simulink model "Simulation"  (Simulink 6.0)
settings: Solver=ode3  StartTime=0.0  StopTime=10  FixedStep=5e-3  RelTol=5e-3
libraries: simulink x40, mblibv1 x14, aerolibtransform2 x5, aerolibutil x5
(part 1 of 2)
settings Model: LastModifiedBy=sebastien
settings OptimizationCC: InlineInvariantSignals=off
settings SimMechanicsCC: VisDuringSimulation=on

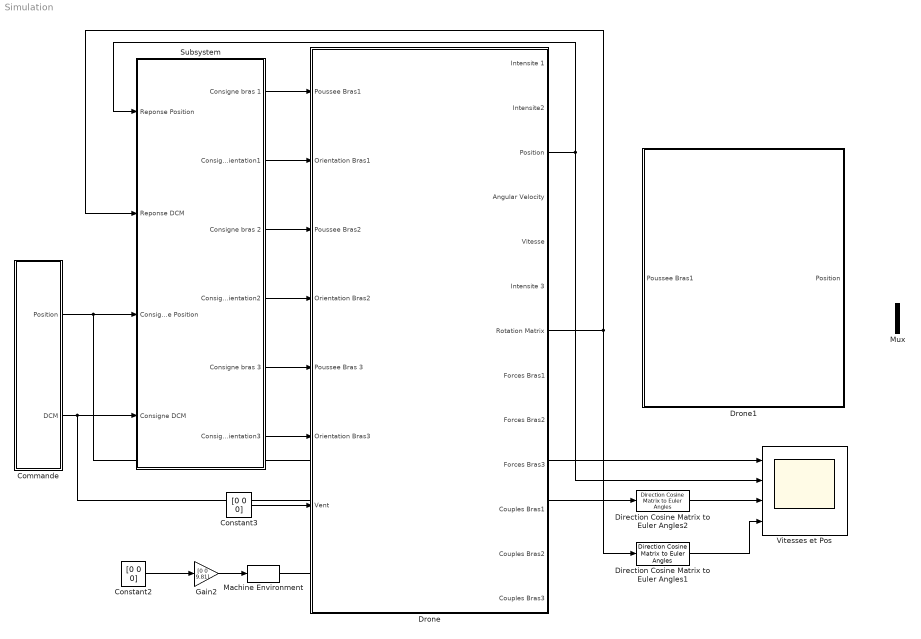
== system Simulation ==
  Commande : Subsystem
  Constant2 : Constant  Value=[0 0 0]
  Constant3 : Constant  Value=[0 0 0]
  Direction Cosine Matrix to Euler Angles1 : aerolibtransform2/Direction Cosine Matrix to Euler Angles
  Direction Cosine Matrix to Euler Angles2 : aerolibtransform2/Direction Cosine Matrix to Euler Angles
  Drone : Subsystem
  Drone1 : Subsystem
  Gain2 : Gain  Gain=[0 0 9.81]
  Machine Environment : mblibv1/Bodies/Machine Environment  Tag=Factory ground  DialogController=MECH.DialogSource  Opaque=on  PortType=env  PhysicalDomain=Mechanical  DialogTemplateClass=MECH.MachineEnvironment  SyncWhenCopied=off  Gravity=[0 0 9.81]  GravityUnits=m/s^2  GravityAsSignal=on  Dimensionality=Auto-detect  AnalysisType=Forward dynamics  LinearAssemblyTolerance=1e-3  LinearAssemblyToleranceUnits=m  AngularAssemblyTolerance=1e-3  AngularAssemblyToleranceUnits=rad  ConstraintSolverType=Stabilizing  ConstraintRelTolerance=1e-4  ConstraintAbsTolerance=1e-4  UseRobustSingularityHandling=off  StatePerturbationType=Fixed  PerturbationSize=1e-5  VisualizeMachine=on
  Mux : Mux  Inputs=2
  Subsystem : Subsystem
  Vitesses et Pos : Scope  NumInputPorts=4
      settings: YMin=-3.5~-45~-9000~-5  YMax=1~5~4000~5  SaveName=ScopeData4
  wires:
  Constant3/1 -> Drone/7(Vent)
  Constant2/1 -> Gain2/1
  Gain2/1 -> Machine Environment/1
  Subsystem/1(Consigne bras 1) -> Drone/1(Poussee Bras1)
  Subsystem/2(Consigne orientation1) -> Drone/2(Orientation Bras1)
  Subsystem/3(Consigne bras 2) -> Drone/3(Poussee Bras2)
  Subsystem/4(Consigne orientation2) -> Drone/4(Orientation Bras2)
  Subsystem/5(Consigne bras 3) -> Drone/5(Poussee Bras 3)
  Subsystem/6(Consigne orientation3) -> Drone/6(Orientation Bras3)
  Drone/7(Rotation Matrix) -> Subsystem/2(Reponse DCM), Direction Cosine Matrix to Euler Angles1/1
  Drone/3(Position) -> Subsystem/1(Reponse Position), Vitesses et Pos/2
  Commande/1(Position) -> Subsystem/3(Consigne Position), Vitesses et Pos/1
  Commande/2(DCM) -> Subsystem/4(Consigne DCM), Direction Cosine Matrix to Euler Angles2/1
  Direction Cosine Matrix to Euler Angles1/1 -> Vitesses et Pos/4
  Direction Cosine Matrix to Euler Angles2/1 -> Vitesses et Pos/3
  connections:
  Drone/LConn1 -- Machine Environment/RConn1

== system Simulation/Commande ==
  Constant : Constant  Value=[0 0 0 0 0 0]
  Demux : Demux  Outputs=2
  Euler Angles to  Direction Cosine Matrix : aerolibtransform2/Euler Angles to  Direction Cosine Matrix
  From File : FromFile  FileName=commande.mat  SampleTime=0
  Reshape1 : simulink/Math Operations/Reshape  OutputDimensionality=1-D array  OutputDimensions=[1,1]
  Reshape2 : simulink/Math Operations/Reshape  OutputDimensionality=1-D array  OutputDimensions=[1,1]
  Reshape3 : simulink/Math Operations/Reshape  OutputDimensionality=1-D array  OutputDimensions=[1,1]
  Position : Outport
  DCM : Outport  Port=2
  wires:
  Reshape2/1 -> Euler Angles to  Direction Cosine Matrix/1
  Reshape3/1 -> Demux/1
  Demux/1 -> Reshape1/1
  Demux/2 -> Reshape2/1
  Reshape1/1 -> Position/1
  From File/1 -> Reshape3/1
  Euler Angles to  Direction Cosine Matrix/1 -> DCM/1

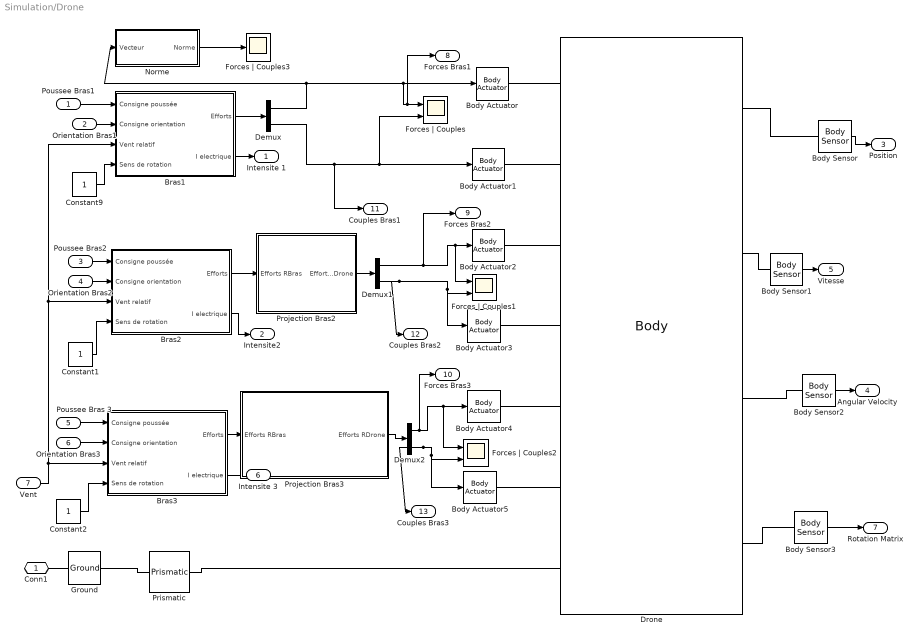
== system Simulation/Drone ==
  Poussee Bras1 : Inport  Port=1  LatchInput=off
  Orientation Bras1 : Inport  Port=2  LatchInput=off
  Poussee Bras2 : Inport  Port=3  LatchInput=off
  Orientation Bras2 : Inport  Port=4  LatchInput=off
  Poussee Bras 3 : Inport  Port=5  LatchInput=off
  Orientation Bras3 : Inport  Port=6  LatchInput=off
  Vent : Inport  Port=7  LatchInput=off
  Body Actuator : mblibv1/Sensors &  Actuators/Body Actuator  Opaque=on  PhysicalDomain=Mechanical  PortType=blob  ActuationStyle=Force  AngleUnits=deg  ArcVelocityUnits=deg/s  ArcAccelerationUnits=deg/s^2  CoordPositionUnits=m  VelocityUnits=m/s  AccelerationUnits=m/s^2  ForceUnits=N  TorqueUnits=N-m  ActiveIO=on  Width=3  DialogClass=MechanicalActuatorBlock  ReferenceFrame=Local (Body CS)  Angle=off  CoordPosition=on  Force=on  Torque=off
  Body Actuator1 : mblibv1/Sensors &  Actuators/Body Actuator  Opaque=on  PhysicalDomain=Mechanical  PortType=blob  ActuationStyle=Force  AngleUnits=deg  ArcVelocityUnits=deg/s  ArcAccelerationUnits=deg/s^2  CoordPositionUnits=m  VelocityUnits=m/s  AccelerationUnits=m/s^2  ForceUnits=N  TorqueUnits=N-m  ActiveIO=on  Width=3  DialogClass=MechanicalActuatorBlock  ReferenceFrame=Local (Body CS)  Angle=off  CoordPosition=on  Force=off  Torque=on
  Body Actuator2 : mblibv1/Sensors &  Actuators/Body Actuator  Opaque=on  PhysicalDomain=Mechanical  PortType=blob  ActuationStyle=Force  AngleUnits=deg  ArcVelocityUnits=deg/s  ArcAccelerationUnits=deg/s^2  CoordPositionUnits=m  VelocityUnits=m/s  AccelerationUnits=m/s^2  ForceUnits=N  TorqueUnits=N-m  ActiveIO=on  Width=3  DialogClass=MechanicalActuatorBlock  ReferenceFrame=Local (Body CS)  Angle=off  CoordPosition=on  Force=on  Torque=off
  Body Actuator3 : mblibv1/Sensors &  Actuators/Body Actuator  Opaque=on  PhysicalDomain=Mechanical  PortType=blob  ActuationStyle=Force  AngleUnits=deg  ArcVelocityUnits=deg/s  ArcAccelerationUnits=deg/s^2  CoordPositionUnits=m  VelocityUnits=m/s  AccelerationUnits=m/s^2  ForceUnits=N  TorqueUnits=N-m  ActiveIO=on  Width=3  DialogClass=MechanicalActuatorBlock  ReferenceFrame=Local (Body CS)  Angle=off  CoordPosition=on  Force=off  Torque=on
  Body Actuator4 : mblibv1/Sensors &  Actuators/Body Actuator  Opaque=on  PhysicalDomain=Mechanical  PortType=blob  ActuationStyle=Force  AngleUnits=deg  ArcVelocityUnits=deg/s  ArcAccelerationUnits=deg/s^2  CoordPositionUnits=m  VelocityUnits=m/s  AccelerationUnits=m/s^2  ForceUnits=N  TorqueUnits=N-m  ActiveIO=on  Width=3  DialogClass=MechanicalActuatorBlock  ReferenceFrame=Local (Body CS)  Angle=off  CoordPosition=on  Force=on  Torque=off
  Body Actuator5 : mblibv1/Sensors &  Actuators/Body Actuator  Opaque=on  PhysicalDomain=Mechanical  PortType=blob  ActuationStyle=Force  AngleUnits=deg  ArcVelocityUnits=deg/s  ArcAccelerationUnits=deg/s^2  CoordPositionUnits=m  VelocityUnits=m/s  AccelerationUnits=m/s^2  ForceUnits=N  TorqueUnits=N-m  ActiveIO=on  Width=3  DialogClass=MechanicalActuatorBlock  ReferenceFrame=Local (Body CS)  Angle=off  CoordPosition=on  Force=off  Torque=on
  Body Sensor : mblibv1/Sensors &  Actuators/Body Sensor  Opaque=on  PhysicalDomain=Mechanical  PortType=blob  Muxed=on  Pose=off  Angle=on  AngleUnits=deg  ArcVelocity=off  ArcVelocityUnits=deg/s  ArcAcceleration=off  ArcAccelerationUnits=deg/s^2  CoordPosition=on  CoordPositionUnits=m  Velocity=off  VelocityUnits=m/s  Acceleration=off  AccelerationUnits=m/s^2  Quaternion=on  QuaternionDT=off  QuaternionDDT=off  OutputVector=[ 3 ]  ActiveIO=on  Width=3  DialogClass=MechanicalSensorBlock  ReferenceFrame=Absolute (World)
  Body Sensor1 : mblibv1/Sensors &  Actuators/Body Sensor  Opaque=on  PhysicalDomain=Mechanical  PortType=blob  Muxed=on  Pose=off  Angle=on  AngleUnits=deg  ArcVelocity=off  ArcVelocityUnits=deg/s  ArcAcceleration=off  ArcAccelerationUnits=deg/s^2  CoordPosition=off  CoordPositionUnits=m  Velocity=on  VelocityUnits=m/s  Acceleration=off  AccelerationUnits=m/s^2  Quaternion=on  QuaternionDT=off  QuaternionDDT=off  QuaternionUnits=off  OutputVector=[ 3 ]  ActiveIO=on  Width=3  DialogClass=MechanicalSensorBlock  ReferenceFrame=Absolute (World)
  Body Sensor2 : mblibv1/Sensors &  Actuators/Body Sensor  Opaque=on  PhysicalDomain=Mechanical  PortType=blob  Muxed=on  Pose=off  Angle=on  AngleUnits=deg  ArcVelocity=on  ArcVelocityUnits=deg/s  ArcAcceleration=off  ArcAccelerationUnits=deg/s^2  CoordPosition=off  CoordPositionUnits=m  Velocity=off  VelocityUnits=m/s  Acceleration=off  AccelerationUnits=m/s^2  Quaternion=on  QuaternionDT=off  QuaternionDDT=off  QuaternionUnits=off  OutputVector=[ 3 ]  ActiveIO=on  Width=3  DialogClass=MechanicalSensorBlock  ReferenceFrame=Absolute (World)
  Body Sensor3 : mblibv1/Sensors &  Actuators/Body Sensor  Opaque=on  PhysicalDomain=Mechanical  PortType=blob  Muxed=on  Pose=on  Angle=on  AngleUnits=deg  ArcVelocity=off  ArcVelocityUnits=deg/s  ArcAcceleration=off  ArcAccelerationUnits=deg/s^2  CoordPosition=off  CoordPositionUnits=m  Velocity=off  VelocityUnits=m/s  Acceleration=off  AccelerationUnits=m/s^2  Quaternion=on  QuaternionDT=off  QuaternionDDT=off  QuaternionUnits=off  OutputVector=[ 9 ]  ActiveIO=on  Width=9  DialogClass=MechanicalSensorBlock  ReferenceFrame=Absolute (World)
  Bras1 : Subsystem
  Bras2 : Subsystem
  Bras3 : Subsystem
  Constant1 : Constant
  Constant2 : Constant
  Constant9 : Constant
  Demux : Demux  Outputs=2
  Demux1 : Demux  Outputs=2
  Demux2 : Demux  Outputs=2
  Drone : mblibv1/Bodies/Body  PhysicalDomain=mechanical  SubClassName=Unknown  LeftPortType=workingframe  RightPortType=workingframe  LConnTagsString=CS3|CS9|CS5|CS10|CS4|CS11|CS1  RConnTagsString=CS2|CS6|CS7|CS8  DialogClass=MechanicalBodyBlock  Mass=1.331  MassUnits=kg  InertiaUnits=kg*m^2  Inertia=[1e-2 9.762e-8 1.027e-6;9.762e-8 0.01 -6.855e-6; 1.027e-6 -6.855e-6 0.018 ]  Shape=Cylinder  ShapeDims=[1 1]  ShapeUnits=m  ShapeUse=false  Density=1  DensityUnits=kg/m^3  DensityUse=false  CG=Left$CG$[0 0 0]$WORLD$WORLD$m$[0 0 0]$Euler X-Y-Z$deg$WORLD$false  WorkingFrames=Right$CS2$[0 0 0]$CG$CG$m$[0 0 0]$Euler X-Y-Z$deg$WORLD$true#Left$CS3$[0.21 0 0]$CG$CG$m$[0 0 0]$Euler X-Y-Z$deg$WORLD$true#Left$CS9$[0.21 0 0]$CG$CG$m$[0 0 0]$Euler X-Y-Z$deg$WORLD$true#Left$CS5$[-0.105 0.1819 0]$CG$CG$m$[0 0 0]$Euler X-Y-Z$deg$WORLD$true#Left$CS10$[-0.105 0.1819 0]$CG$CG$m$[0 0 0]$Euler X-Y-Z$deg$WORLD$true#Left$CS4$[-0.105 -0.1819 0]$CG$CG$m$[0 0 0]$Euler X-Y-Z$deg$WORLD$true#Left$CS11$[-0.105 -0.1819 0]$CG$CG$m$[0 0 0]$Euler X-Y-Z$deg$WORLD$true#Right$CS6$[0 0 0]$CG$CG$m$[0 0 0]$Euler X-Y-Z$deg$WORLD$true#Right$CS7$[0 0 0]$CG$CG$m$[0 0 0]$Euler X-Y-Z$deg$WORLD$true#Right$CS8$[0 0 0]$CG$CG$m$[0 0 0]$Euler X-Y-Z$deg$WORLD$true#Left$CS1$[0 0 0]$CG$CG$m$[0 0 0]$Euler X-Y-Z$deg$WORLD$true
  Forces | Couples : Scope  NumInputPorts=2
      settings: YMin=-6~-1.5  YMax=4~0
  Forces | Couples1 : Scope  NumInputPorts=2
      settings: YMin=-4~-1.25  YMax=0.5~0
  Forces | Couples2 : Scope  NumInputPorts=2
      settings: YMin=-6~-1.5  YMax=1~1.25  SaveName=ScopeData2
  Forces | Couples3 : Scope
      settings: YMin=0  YMax=5.5  SaveName=ScopeData16
  Ground : mblibv1/Bodies/Ground  Opaque=on  LeftPortType=env  RightPortType=workingframe  PhysicalDomain=Mechanical  DialogClass=GroundBlock  CoordPosition=[0 0 0]  CoordPositionUnits=m  StateVectorMgrId=-1  MachineId=[1 0]  ShowEnvPort=on
  Norme : Subsystem  mask{ordre=2}
      mask Display: text(0.3,0.5,strcat('Norme',get_param(gcb, 'ordre')));
  Prismatic : mblibv1/Joints/Prismatic  PhysicalDomain=mechanical  SubClassName=Unknown  LeftPortType=blob  RightPortType=blob  LConnTagsString=__newl0  RConnTagsString=__newr0  NumSAPorts=0  CutJoint=off  MarkAsCut=off  Primitives=prismatic  PrimitiveProps=P1$WORLD$[0 0 1]$prismatic  DialogClass=JointBlock
  Projection Bras2 : Subsystem
  Projection Bras3 : Subsystem
  Conn1 : PMIOPort  Port=1  Side=Left
  Intensite 1 : Outport
  Intensite2 : Outport  Port=2
  Position : Outport  Port=3
  Angular Velocity : Outport  Port=4
  Vitesse : Outport  Port=5
  Intensite 3 : Outport  Port=6
  Rotation Matrix : Outport  Port=7
  Forces Bras1 : Outport  Port=8
  Forces Bras2 : Outport  Port=9
  Forces Bras3 : Outport  Port=10
  Couples Bras1 : Outport  Port=11
  Couples Bras2 : Outport  Port=12
  Couples Bras3 : Outport  Port=13
  wires:
  Bras1/1(Efforts) -> Demux/1
  Demux/1 -> Body Actuator/1, Forces | Couples/1, Forces Bras1/1, Norme/1(Vecteur)
  Demux/2 -> Body Actuator1/1, Forces | Couples/2, Couples Bras1/1
  Bras2/1(Efforts) -> Projection Bras2/1(Efforts RBras)
  Demux1/1 -> Body Actuator2/1, Forces | Couples1/1, Forces Bras2/1
  Demux1/2 -> Body Actuator3/1, Forces | Couples1/2, Couples Bras2/1
  Projection Bras2/1(Efforts RDrone) -> Demux1/1
  Bras3/1(Efforts) -> Projection Bras3/1(Efforts RBras)
  Demux2/1 -> Body Actuator4/1, Forces | Couples2/1, Forces Bras3/1
  Demux2/2 -> Body Actuator5/1, Forces | Couples2/2, Couples Bras3/1
  Projection Bras3/1(Efforts RDrone) -> Demux2/1
  Poussee Bras 3/1 -> Bras3/1(Consigne poussée)
  Constant9/1 -> Bras1/4(Sens de rotation)
  Poussee Bras1/1 -> Bras1/1(Consigne poussée)
  Orientation Bras1/1 -> Bras1/2(Consigne orientation)
  Bras1/2(I electrique) -> Intensite 1/1
  Poussee Bras2/1 -> Bras2/1(Consigne poussée)
  Orientation Bras2/1 -> Bras2/2(Consigne orientation)
  Bras2/2(I electrique) -> Intensite2/1
  Body Sensor/1 -> Position/1
  Body Sensor2/1 -> Angular Velocity/1
  Orientation Bras3/1 -> Bras3/2(Consigne orientation)
  Body Sensor1/1 -> Vitesse/1
  Bras3/2(I electrique) -> Intensite 3/1
  Vent/1 -> Bras1/3(Vent relatif), Bras2/3(Vent relatif), Bras3/3(Vent relatif)
  Body Sensor3/1 -> Rotation Matrix/1
  Constant2/1 -> Bras3/4(Sens de rotation)
  Constant1/1 -> Bras2/4(Sens de rotation)
  Norme/1(Norme) -> Forces | Couples3/1
  connections:
  Body Actuator/RConn1 -- Drone/LConn1
  Body Actuator1/RConn1 -- Drone/LConn2
  Body Actuator2/RConn1 -- Drone/LConn3
  Body Actuator3/RConn1 -- Drone/LConn4
  Body Actuator4/RConn1 -- Drone/LConn5
  Body Actuator5/RConn1 -- Drone/LConn6
  Body Sensor/LConn1 -- Drone/RConn1
  Body Sensor1/LConn1 -- Drone/RConn2
  Drone/RConn3 -- Body Sensor2/LConn1
  Body Sensor3/LConn1 -- Drone/RConn4
  Prismatic/RConn1 -- Drone/LConn7
  Ground/RConn1 -- Prismatic/LConn1
  Conn1/RConn1 -- Ground/LConn1

== system Simulation/Drone1 ==
  Poussee Bras1 : Inport  Port=1  LatchInput=off
  Bras1 : Subsystem  mask{sens=0}
      mask prompts: sens "Sens de rotation"
  Position : Outport

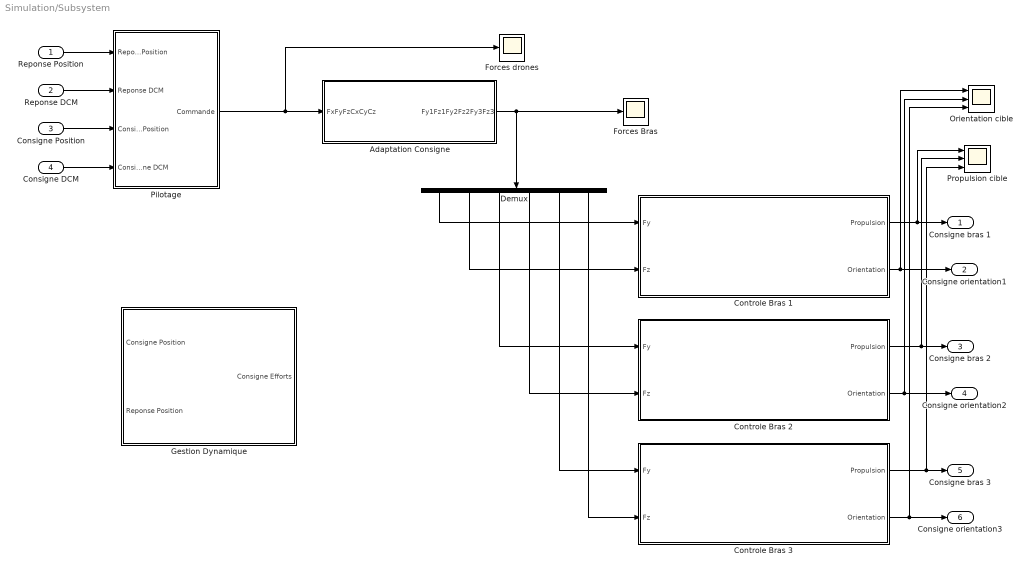
== system Simulation/Subsystem ==
  Reponse Position : Inport  Port=1  LatchInput=off
  Reponse DCM : Inport  Port=2  LatchInput=off
  Consigne Position : Inport  Port=3  LatchInput=off
  Consigne DCM : Inport  Port=4  LatchInput=off
  Adaptation Consigne : Subsystem  mask{l=0.21}
      mask prompts: l "Longueur Bras"
  Controle Bras 1 : Subsystem
  Controle Bras 2 : Subsystem
  Controle Bras 3 : Subsystem
  Demux : Demux  Orientation=down  Outputs=6
  Forces Bras : Scope
      settings: YMin=-0.24  YMax=2.77556e-017  SaveName=ScopeData14
  Forces drones : Scope
      settings: YMin=-0.75  YMax=0  SaveName=ScopeData5
  Gestion Dynamique : Subsystem
  Orientation cible : Scope  NumInputPorts=3
      settings: YMin=-3.5~-5~-5  YMax=3.5~5~5  SaveName=ScopeData15
  Pilotage : Subsystem
  Propulsion cible : Scope  NumInputPorts=3
      settings: YMin=1.9~0~-5  YMax=2.1~2~5  SaveName=ScopeData9
  Consigne bras 1 : Outport
  Consigne orientation1 : Outport  Port=2
  Consigne bras 2 : Outport  Port=3
  Consigne orientation2 : Outport  Port=4
  Consigne bras 3 : Outport  Port=5
  Consigne orientation3 : Outport  Port=6
  wires:
  Pilotage/1(Commande) -> Adaptation Consigne/1(FxFyFzCxCyCz), Forces drones/1
  Reponse Position/1 -> Pilotage/1(Reponse Position)
  Reponse DCM/1 -> Pilotage/2(Reponse DCM)
  Demux/1 -> Controle Bras 1/1(Fy)
  Demux/2 -> Controle Bras 1/2(Fz)
  Adaptation Consigne/1(Fy1Fz1Fy2Fz2Fy3Fz3) -> Demux/1, Forces Bras/1
  Demux/3 -> Controle Bras 2/1(Fy)
  Demux/4 -> Controle Bras 2/2(Fz)
  Demux/5 -> Controle Bras 3/1(Fy)
  Demux/6 -> Controle Bras 3/2(Fz)
  Consigne Position/1 -> Pilotage/3(Consigne Position)
  Consigne DCM/1 -> Pilotage/4(Consigne DCM)
  Controle Bras 1/1(Propulsion) -> Consigne bras 1/1, Propulsion cible/1
  Controle Bras 1/2(Orientation) -> Consigne orientation1/1, Orientation cible/1
  Controle Bras 2/1(Propulsion) -> Consigne bras 2/1, Propulsion cible/2
  Controle Bras 2/2(Orientation) -> Consigne orientation2/1, Orientation cible/2
  Controle Bras 3/1(Propulsion) -> Consigne bras 3/1, Propulsion cible/3
  Controle Bras 3/2(Orientation) -> Consigne orientation3/1, Orientation cible/3

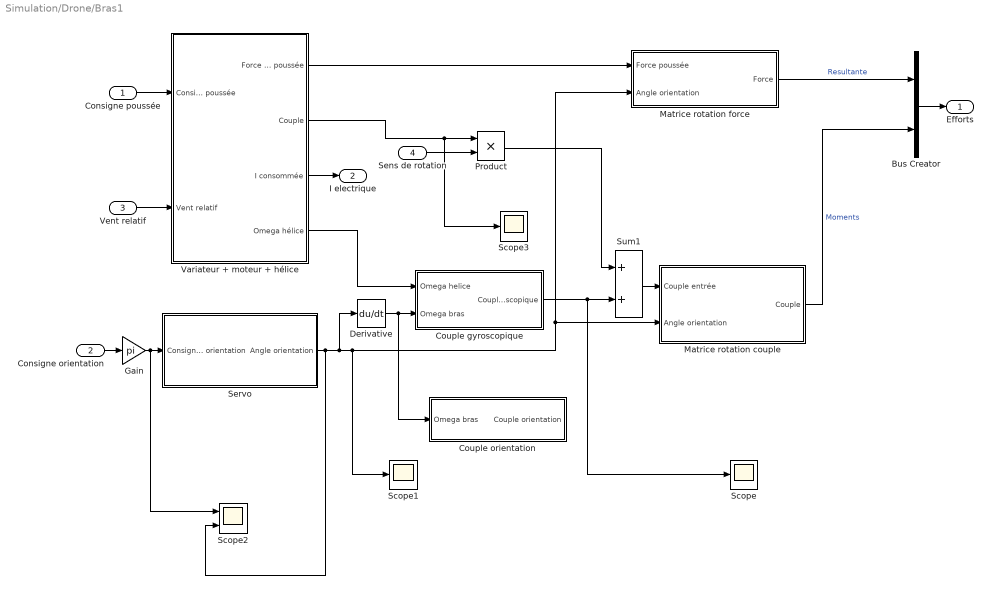
== system Simulation/Drone/Bras1 ==
  Consigne poussée : Inport  Port=1  LatchInput=off
  Consigne orientation : Inport  Port=2  LatchInput=off
  Vent relatif : Inport  Port=3  LatchInput=off
  Sens de rotation : Inport  Port=4  LatchInput=off
  " Couple orientation" : Subsystem
  Bus Creator : BusCreator  DialogController=Simulink.DDGSource_Bus  Inputs=2
  Couple gyroscopique : Subsystem
  Derivative : Derivative
  Gain : Gain  Gain=pi
  Matrice rotation couple : Subsystem
  Matrice rotation force : Subsystem
  Product : Product  RndMeth=Zero
  Scope : Scope
      settings: YMin=-1  YMax=1  SaveName=ScopeData3
  Scope1 : Scope
      settings: YMin=-0.5  YMax=3.75  SaveName=ScopeData8
  Scope2 : Scope  NumInputPorts=2
      settings: YMin=-3~-5  YMax=3~5  SaveName=ScopeData12
  Scope3 : Scope
      settings: YMin=-1  YMax=1  SaveName=ScopeData13
  Servo : Subsystem
  Sum1 : Sum
  Variateur + moteur + hélice : Subsystem
  Efforts : Outport
  I electrique : Outport  Port=2
  wires:
  Consigne poussée/1 -> Variateur + moteur + hélice/1(Consigne poussée)
  Servo/1(Angle orientation) -> Derivative/1, Matrice rotation force/2(Angle orientation), Matrice rotation couple/2(Angle orientation), Scope1/1, Scope2/2
  Matrice rotation force/1(Force) -> Bus Creator/1  "Resultante"
  Matrice rotation couple/1(Couple) -> Bus Creator/2  "Moments"
  Derivative/1 -> Couple gyroscopique/2(Omega bras), " Couple orientation"/1(Omega bras)
  Sum1/1 -> Matrice rotation couple/1(Couple entrée)
  Couple gyroscopique/1(Couple gyroscopique) -> Sum1/2, Scope/1
  Bus Creator/1 -> Efforts/1
  Consigne orientation/1 -> Gain/1
  Vent relatif/1 -> Variateur + moteur + hélice/2(Vent relatif)
  Variateur + moteur + hélice/1(Force de poussée) -> Matrice rotation force/1(Force poussée)
  Variateur + moteur + hélice/3(I consommée) -> I electrique/1
  Variateur + moteur + hélice/4(Omega hélice) -> Couple gyroscopique/1(Omega helice)
  Gain/1 -> Servo/1(Consigne orientation), Scope2/1
  Sens de rotation/1 -> Product/2
  Product/1 -> Sum1/1
  Variateur + moteur + hélice/2(Couple) -> Product/1, Scope3/1

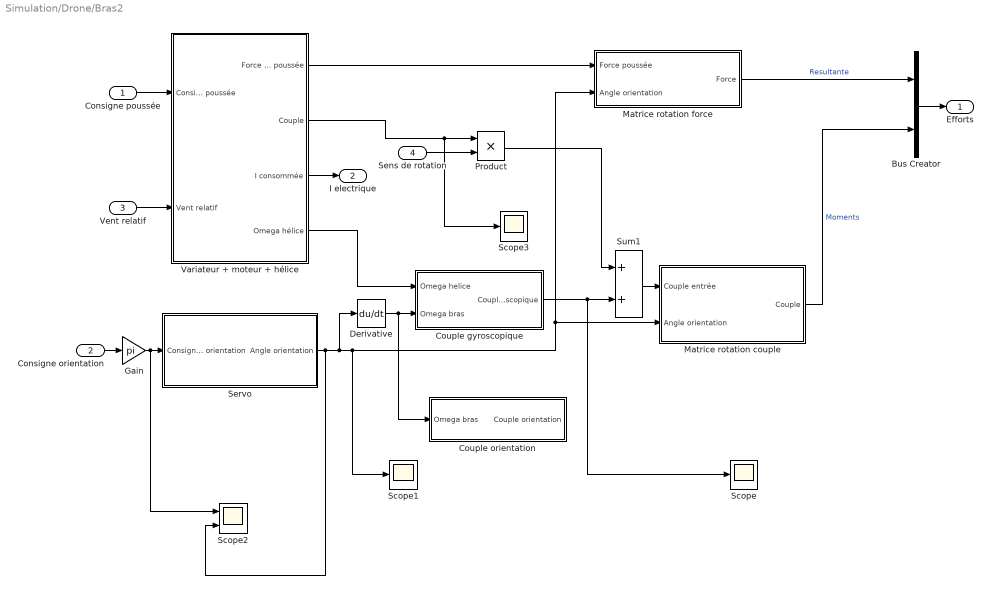
== system Simulation/Drone/Bras2 ==
  Consigne poussée : Inport  Port=1  LatchInput=off
  Consigne orientation : Inport  Port=2  LatchInput=off
  Vent relatif : Inport  Port=3  LatchInput=off
  Sens de rotation : Inport  Port=4  LatchInput=off
  " Couple orientation" : Subsystem
  Bus Creator : BusCreator  DialogController=Simulink.DDGSource_Bus  Inputs=2
  Couple gyroscopique : Subsystem
  Derivative : Derivative
  Gain : Gain  Gain=pi
  Matrice rotation couple : Subsystem
  Matrice rotation force : Subsystem
  Product : Product  RndMeth=Zero
  Scope : Scope
      settings: YMin=-1  YMax=1  SaveName=ScopeData3
  Scope1 : Scope
      settings: YMin=-2.85  YMax=-2.15  SaveName=ScopeData8
  Scope2 : Scope  NumInputPorts=2
      settings: YMin=-3~-5  YMax=3~5  SaveName=ScopeData12
  Scope3 : Scope
      settings: YMin=-1  YMax=1  SaveName=ScopeData13
  Servo : Subsystem
  Sum1 : Sum
  Variateur + moteur + hélice : Subsystem
  Efforts : Outport
  I electrique : Outport  Port=2
  wires:
  Consigne poussée/1 -> Variateur + moteur + hélice/1(Consigne poussée)
  Servo/1(Angle orientation) -> Derivative/1, Matrice rotation force/2(Angle orientation), Matrice rotation couple/2(Angle orientation), Scope1/1, Scope2/2
  Matrice rotation force/1(Force) -> Bus Creator/1  "Resultante"
  Matrice rotation couple/1(Couple) -> Bus Creator/2  "Moments"
  Derivative/1 -> Couple gyroscopique/2(Omega bras), " Couple orientation"/1(Omega bras)
  Sum1/1 -> Matrice rotation couple/1(Couple entrée)
  Couple gyroscopique/1(Couple gyroscopique) -> Sum1/2, Scope/1
  Bus Creator/1 -> Efforts/1
  Consigne orientation/1 -> Gain/1
  Vent relatif/1 -> Variateur + moteur + hélice/2(Vent relatif)
  Variateur + moteur + hélice/1(Force de poussée) -> Matrice rotation force/1(Force poussée)
  Variateur + moteur + hélice/3(I consommée) -> I electrique/1
  Variateur + moteur + hélice/4(Omega hélice) -> Couple gyroscopique/1(Omega helice)
  Gain/1 -> Servo/1(Consigne orientation), Scope2/1
  Sens de rotation/1 -> Product/2
  Product/1 -> Sum1/1
  Variateur + moteur + hélice/2(Couple) -> Product/1, Scope3/1

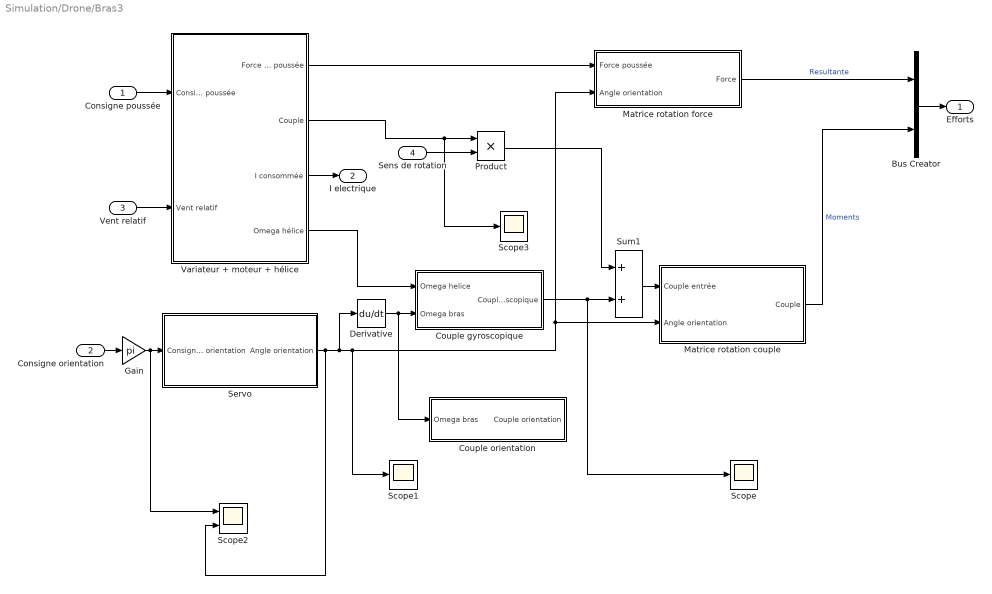
== system Simulation/Drone/Bras3 ==
  Consigne poussée : Inport  Port=1  LatchInput=off
  Consigne orientation : Inport  Port=2  LatchInput=off
  Vent relatif : Inport  Port=3  LatchInput=off
  Sens de rotation : Inport  Port=4  LatchInput=off
  " Couple orientation" : Subsystem
  Bus Creator : BusCreator  DialogController=Simulink.DDGSource_Bus  Inputs=2
  Couple gyroscopique : Subsystem
  Derivative : Derivative
  Gain : Gain  Gain=pi
  Matrice rotation couple : Subsystem
  Matrice rotation force : Subsystem
  Product : Product  RndMeth=Zero
  Scope : Scope
      settings: YMin=-1  YMax=1  SaveName=ScopeData3
  Scope1 : Scope
      settings: YMin=-2.85  YMax=-2.15  SaveName=ScopeData8
  Scope2 : Scope  NumInputPorts=2
      settings: YMin=-3~-5  YMax=3~5  SaveName=ScopeData12
  Scope3 : Scope
      settings: YMin=-1  YMax=1  SaveName=ScopeData13
  Servo : Subsystem
  Sum1 : Sum
  Variateur + moteur + hélice : Subsystem
  Efforts : Outport
  I electrique : Outport  Port=2
  wires:
  Consigne poussée/1 -> Variateur + moteur + hélice/1(Consigne poussée)
  Servo/1(Angle orientation) -> Derivative/1, Matrice rotation force/2(Angle orientation), Matrice rotation couple/2(Angle orientation), Scope1/1, Scope2/2
  Matrice rotation force/1(Force) -> Bus Creator/1  "Resultante"
  Matrice rotation couple/1(Couple) -> Bus Creator/2  "Moments"
  Derivative/1 -> Couple gyroscopique/2(Omega bras), " Couple orientation"/1(Omega bras)
  Sum1/1 -> Matrice rotation couple/1(Couple entrée)
  Couple gyroscopique/1(Couple gyroscopique) -> Sum1/2, Scope/1
  Bus Creator/1 -> Efforts/1
  Consigne orientation/1 -> Gain/1
  Vent relatif/1 -> Variateur + moteur + hélice/2(Vent relatif)
  Variateur + moteur + hélice/1(Force de poussée) -> Matrice rotation force/1(Force poussée)
  Variateur + moteur + hélice/3(I consommée) -> I electrique/1
  Variateur + moteur + hélice/4(Omega hélice) -> Couple gyroscopique/1(Omega helice)
  Gain/1 -> Servo/1(Consigne orientation), Scope2/1
  Sens de rotation/1 -> Product/2
  Product/1 -> Sum1/1
  Variateur + moteur + hélice/2(Couple) -> Product/1, Scope3/1

== system Simulation/Drone/Norme ==
  Vecteur : Inport  Port=1  LatchInput=off
  Constant1 : Constant  Value=ordre
  Math Function : Math  Operator=pow  SaturateOnIntegerOverflow=on
  Math Function1 : Math  Operator=reciprocal  SaturateOnIntegerOverflow=on
  Math Function2 : Math  Operator=pow  SaturateOnIntegerOverflow=on
  Sum of Elements : Sum  Inputs=+  OutScaling=2^-10
  Norme : Outport
  wires:
  Math Function/1 -> Sum of Elements/1
  Vecteur/1 -> Math Function/1
  Constant1/1 -> Math Function/2, Math Function1/1
  Math Function1/1 -> Math Function2/2
  Sum of Elements/1 -> Math Function2/1
  Math Function2/1 -> Norme/1

== system Simulation/Drone/Projection Bras2 ==
  note: Forces
  note: Moments
  Efforts RBras : Inport  Port=1  LatchInput=off
  Bus Creator : BusCreator  DialogController=Simulink.DDGSource_Bus  Inputs=2
  Demux : Demux  Outputs=2
  Gain : Gain  Gain=[cos(2*pi/3) -sin(2*pi/3) 0 ; sin(2*pi/3) cos(2*pi/3) 0; 0 0 1]  Multiplication=Matrix(K*u) (u vector)
  Gain1 : Gain  Gain=[cos(2*pi/3) -sin(2*pi/3) 0 ; sin(2*pi/3) cos(2*pi/3) 0; 0 0 1]  Multiplication=Matrix(K*u) (u vector)
  Efforts RDrone : Outport
  wires:
  Efforts RBras/1 -> Demux/1
  Demux/1 -> Gain/1
  Demux/2 -> Gain1/1
  Bus Creator/1 -> Efforts RDrone/1
  Gain/1 -> Bus Creator/1
  Gain1/1 -> Bus Creator/2

== system Simulation/Drone/Projection Bras3 ==
  note: Forces
  note: Moments
  Efforts RBras : Inport  Port=1  LatchInput=off
  Bus Creator : BusCreator  DialogController=Simulink.DDGSource_Bus  Inputs=2
  Demux : Demux  Outputs=2
  Matrice de Rotation : Gain  Gain=[cos(4*pi/3) -sin(4*pi/3) 0 ; sin(4*pi/3) cos(4*pi/3) 0; 0 0 1]  Multiplication=Matrix(K*u) (u vector)
  "Matrice de rotation " : Gain  Gain=[cos(4*pi/3) -sin(4*pi/3) 0 ; sin(4*pi/3) cos(4*pi/3) 0; 0 0 1]  Multiplication=Matrix(K*u) (u vector)
  Efforts RDrone : Outport
  wires:
  Efforts RBras/1 -> Demux/1
  Demux/1 -> Matrice de Rotation/1
  Demux/2 -> "Matrice de rotation "/1
  Bus Creator/1 -> Efforts RDrone/1
  Matrice de Rotation/1 -> Bus Creator/1
  "Matrice de rotation "/1 -> Bus Creator/2

== system Simulation/Drone1/Bras1 ==
  Consigne poussée : Inport  Port=1  LatchInput=off
  Consigne orientation : Inport  Port=2  LatchInput=off
  Vent relatif : Inport  Port=3  LatchInput=off
  " Couple orientation" : Subsystem
  Bus Creator : BusCreator  DialogController=Simulink.DDGSource_Bus  Inputs=2
  Constant : Constant  Value=sens
  Couple gyroscopique : Subsystem
  Derivative : Derivative
  Gain : Gain  Gain=pi
  Matrice rotation couple : Subsystem
  Matrice rotation force : Subsystem
  Product : Product  RndMeth=Zero
  Servo : Subsystem
  Sum1 : Sum  Inputs=+++
  Variateur + moteur + hélice : Subsystem
  Efforts : Outport
  I electrique : Outport  Port=2
  wires:
  Consigne poussée/1 -> Variateur + moteur + hélice/1(Consigne poussée)
  Servo/1(Angle orientation) -> Derivative/1, Matrice rotation force/2(Angle orientation), Matrice rotation couple/2(Angle orientation)
  Matrice rotation force/1(Force) -> Bus Creator/1  "Resultante"
  Matrice rotation couple/1(Couple) -> Bus Creator/2  "Moments"
  Derivative/1 -> Couple gyroscopique/2(Omega bras), " Couple orientation"/1(Omega bras)
  Sum1/1 -> Matrice rotation couple/1(Couple entrée)
  Couple gyroscopique/1(Couple gyroscopique) -> Sum1/2
  Bus Creator/1 -> Efforts/1
  Consigne orientation/1 -> Gain/1
  Vent relatif/1 -> Variateur + moteur + hélice/2(Vent relatif)
  Variateur + moteur + hélice/1(Force de poussée) -> Matrice rotation force/1(Force poussée)
  Variateur + moteur + hélice/3(I consommée) -> I electrique/1
  Variateur + moteur + hélice/4(Omega hélice) -> Couple gyroscopique/1(Omega helice)
  Gain/1 -> Servo/1(Consigne orientation)
  Constant/1 -> Product/2
  Product/1 -> Sum1/1
  Variateur + moteur + hélice/2(Couple) -> Product/1
  " Couple orientation"/1(Couple orientation) -> Sum1/3

== system Simulation/Subsystem/Adaptation Consigne ==
  FxFyFzCxCyCz : Inport  Port=1  LatchInput=off
  Matrice Correction : Constant  Value=[1 1 1 1/l 1/l 1/l]
  Matrice Transformation : Constant  Value=(1/3)*[0 2 0 0 0 1; 0 0 1 0 2 0; -sqrt(3) -1 0 0 0 1; 0 0 1 -sqrt(3) -1 0; sqrt(3) -1 0 0 0 1; 0 0 1 sqrt(3) -1 0]  VectorParams1D=off
  Product : Product  Multiplication=Matrix(*)  RndMeth=Zero
  Product1 : Product  RndMeth=Zero
  Fy1Fz1Fy2Fz2Fy3Fz3 : Outport
  wires:
  Product/1 -> Fy1Fz1Fy2Fz2Fy3Fz3/1
  Matrice Transformation/1 -> Product/1
  Matrice Correction/1 -> Product1/2
  FxFyFzCxCyCz/1 -> Product1/1
  Product1/1 -> Product/2

== system Simulation/Subsystem/Controle Bras 1 ==
  Fy : Inport  Port=1  LatchInput=off
  Fz : Inport  Port=2  LatchInput=off
  Adaptation Consigne1 : Subsystem  mask{a=2e-5, b=1e-3, c=2e-3}
  Controle Bras1 : Subsystem
  Gain : Gain  Gain=60/(500*2*pi)
  Gain5 : Gain  Gain=1/pi
  Saturation : Saturate  UpperLimit=pi/6  LowerLimit=-pi/6
  Saturation1 : Saturate  UpperLimit=2  LowerLimit=0
  Saturation6 : Saturate  UpperLimit=1000  LowerLimit=0
  Propulsion : Outport
  Orientation : Outport  Port=2
  wires:
  Controle Bras1/1(Force Propulsion) -> Saturation6/1
  Adaptation Consigne1/1(Consigne Omega) -> Gain/1
  Gain/1 -> Saturation1/1
  Saturation6/1 -> Adaptation Consigne1/1(Force)
  Fy/1 -> Controle Bras1/1(Fyc)
  Saturation1/1 -> Propulsion/1
  Fz/1 -> Controle Bras1/2(Fzc)
  Gain5/1 -> Orientation/1
  Controle Bras1/2(Angle Orientation) -> Gain5/1

== system Simulation/Subsystem/Controle Bras 2 ==
  Fy : Inport  Port=1  LatchInput=off
  Fz : Inport  Port=2  LatchInput=off
  Adaptation Consigne1 : Subsystem  mask{a=2e-5, b=1e-3, c=2e-3}
  Controle Bras1 : Subsystem
  Gain : Gain  Gain=60/(500*2*pi)
  Gain5 : Gain  Gain=1/pi
  Saturation1 : Saturate  UpperLimit=2  LowerLimit=0
  Saturation6 : Saturate  UpperLimit=1000  LowerLimit=0
  Propulsion : Outport
  Orientation : Outport  Port=2
  wires:
  Controle Bras1/1(Force Propulsion) -> Saturation6/1
  Adaptation Consigne1/1(Consigne Omega) -> Gain/1
  Gain/1 -> Saturation1/1
  Saturation6/1 -> Adaptation Consigne1/1(Force)
  Fy/1 -> Controle Bras1/1(Fyc)
  Saturation1/1 -> Propulsion/1
  Fz/1 -> Controle Bras1/2(Fzc)
  Gain5/1 -> Orientation/1
  Controle Bras1/2(Angle Orientation) -> Gain5/1

== system Simulation/Subsystem/Controle Bras 3 ==
  Fy : Inport  Port=1  LatchInput=off
  Fz : Inport  Port=2  LatchInput=off
  Adaptation Consigne1 : Subsystem  mask{a=2e-5, b=1e-3, c=2e-3}
  Controle Bras1 : Subsystem
  Gain : Gain  Gain=60/(500*2*pi)
  Gain5 : Gain  Gain=1/pi
  Saturation1 : Saturate  UpperLimit=2  LowerLimit=0
  Saturation6 : Saturate  UpperLimit=1000  LowerLimit=0
  Propulsion : Outport
  Orientation : Outport  Port=2
  wires:
  Controle Bras1/1(Force Propulsion) -> Saturation6/1
  Adaptation Consigne1/1(Consigne Omega) -> Gain/1
  Gain/1 -> Saturation1/1
  Saturation6/1 -> Adaptation Consigne1/1(Force)
  Fy/1 -> Controle Bras1/1(Fyc)
  Saturation1/1 -> Propulsion/1
  Fz/1 -> Controle Bras1/2(Fzc)
  Gain5/1 -> Orientation/1
  Controle Bras1/2(Angle Orientation) -> Gain5/1

== system Simulation/Subsystem/Gestion Dynamique ==
  Consigne Position : Inport  Port=1  LatchInput=off
  Reponse Position : Inport  Port=2  LatchInput=off
  Calcul Position : Subsystem
  Calcul orientation : Subsystem
  PID Attitude : Subsystem  mask{kp=0.00000000001, ki=0, kd=0, kdd=0}
  PID Position : Subsystem  mask{kp=0.5, ki=0.2, kd=2, kdd=0.3}
  Separation composantes : Subsystem
  Separation composantes1 : Subsystem
  Sommation ordres : Subsystem
  Terminator : Terminator
  Consigne Efforts : Outport
  wires:
  Reponse Position/1 -> Separation composantes1/1(Entree), Separation composantes/2(Reponse1)
  Separation composantes1/2(Orientation) -> Calcul Position/2(Orientation), Calcul orientation/2(Orientation)
  Sommation ordres/1(Ordres) -> Consigne Efforts/1
  Separation composantes1/1(Position) -> Terminator/1
  PID Position/1(Sortie) -> Calcul Position/1(Erreur Position)
  Calcul Position/1(Ordres Position) -> Sommation ordres/1(Ordres position)
  Calcul orientation/1(Ordres orientation) -> Sommation ordres/2(Ordres orientation)
  PID Attitude/1(Sortie) -> Calcul orientation/1(Erreur orientation)
  Consigne Position/1 -> Separation composantes/1(Consigne1)
  Separation composantes/1(Erreur Position) -> PID Position/1(Entrée)
  Separation composantes/2(Erreur Attitude) -> PID Attitude/1(Entrée)

== system Simulation/Subsystem/Pilotage ==
  Reponse Position : Inport  Port=1  LatchInput=off
  Reponse DCM : Inport  Port=2  LatchInput=off
  Consigne Position : Inport  Port=3  LatchInput=off
  Consigne DCM : Inport  Port=4  LatchInput=off
  Add : Sum  Inputs=-+  OutScaling=2^-10  InputSameDT=on
  Attitude : Subsystem
  Multiplication : Product  Inputs=**  Multiplication=Matrix(*)  OutScaling=2^-10
  Multiplication1 : Product  Inputs=**  Multiplication=Matrix(*)  OutScaling=2^-10
  Mux1 : Mux  Inputs=2
  PID Attitude : Subsystem  mask{kp=1000, ki=0.05, kd=0.05, kdd=0}
  PID Position : Subsystem  mask{kp=1000, ki=0.05, kd=0.05, kdd=0}
  Commande : Outport
  wires:
  Reponse Position/1 -> Add/1
  Consigne Position/1 -> Add/2
  Add/1 -> PID Position/1(Entrée)
  Consigne DCM/1 -> Attitude/2(Consigne)
  Reponse DCM/1 -> Attitude/1(Reponse), Multiplication1/1, Multiplication/1
  Attitude/1(Commande) -> PID Attitude/1(Entrée)
  PID Attitude/1(Sortie) -> Multiplication/2
  PID Position/1(Sortie) -> Multiplication1/2
  Multiplication1/1 -> Mux1/1
  Multiplication/1 -> Mux1/2
  Mux1/1 -> Commande/1

== system Simulation/Drone/Bras1/ Couple orientation ==
  Omega bras : Inport  Port=1  LatchInput=off
  Derivative1 : Derivative
  Gain : Gain
  Couple orientation : Outport
  wires:
  Omega bras/1 -> Derivative1/1
  Derivative1/1 -> Gain/1
  Gain/1 -> Couple orientation/1

== system Simulation/Drone/Bras1/Couple gyroscopique ==
  Omega helice : Inport  Port=1  LatchInput=off
  Omega bras : Inport  Port=2  LatchInput=off
  Gain : Gain  Gain=[0 27e-6 0]
  Product : Product  RndMeth=Zero
  Couple gyroscopique : Outport
  wires:
  Omega helice/1 -> Product/1
  Omega bras/1 -> Product/2
  Product/1 -> Gain/1
  Gain/1 -> Couple gyroscopique/1

== system Simulation/Drone/Bras1/Matrice rotation couple ==
  Couple entrée : Inport  Port=1  LatchInput=off
  Angle orientation : Inport  Port=2  LatchInput=off
  Constant : Constant  Value=0
  Cos : Trigonometry  Operator=cos
  Gain : Gain  Gain=[ 1 1 -1 ]
  Mux : Mux  Inputs=3
  Product : Product  RndMeth=Zero
  Reshape : simulink/Math Operations/Reshape  OutputDimensionality=1-D array  OutputDimensions=[1,1]
  Sin : Trigonometry
  Couple : Outport
  wires:
  Angle orientation/1 -> Cos/1, Sin/1
  Constant/1 -> Mux/1
  Cos/1 -> Mux/3
  Sin/1 -> Mux/2
  Mux/1 -> Reshape/1
  Gain/1 -> Product/1
  Couple entrée/1 -> Product/2
  Product/1 -> Couple/1
  Reshape/1 -> Gain/1

== system Simulation/Drone/Bras1/Matrice rotation force ==
  Force poussée : Inport  Port=1  LatchInput=off
  Angle orientation : Inport  Port=2  LatchInput=off
  Constant : Constant  Value=0
  Cos : Trigonometry  Operator=cos
  Gain : Gain  Gain=[ 1 1 -1 ]
  Mux : Mux  Inputs=3
  Product : Product  RndMeth=Zero
  Reshape : simulink/Math Operations/Reshape  OutputDimensionality=1-D array  OutputDimensions=[1,1]
  Sin : Trigonometry
  Force : Outport
  wires:
  Angle orientation/1 -> Cos/1, Sin/1
  Constant/1 -> Mux/1
  Cos/1 -> Mux/3
  Sin/1 -> Mux/2
  Mux/1 -> Reshape/1
  Gain/1 -> Product/1
  Force poussée/1 -> Product/2
  Product/1 -> Force/1
  Reshape/1 -> Gain/1

== system Simulation/Drone/Bras1/Servo ==
  Consigne orientation : Inport  Port=1  LatchInput=off
  Temps de réponse orientation1 : TransferFcn  Denominator=[ 0.002 0.05 1]
  Angle orientation : Outport
  wires:
  Consigne orientation/1 -> Temps de réponse orientation1/1
  Temps de réponse orientation1/1 -> Angle orientation/1

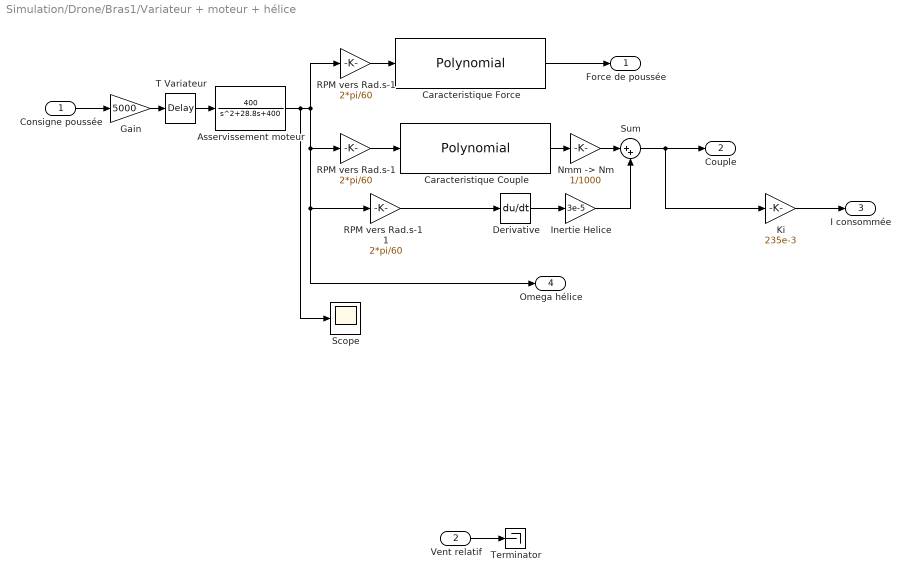
== system Simulation/Drone/Bras1/Variateur + moteur + hélice ==
  Consigne poussée : Inport  Port=1  LatchInput=off
  Vent relatif : Inport  Port=2  LatchInput=off
  Asservissement moteur : TransferFcn  Numerator=[400]  Denominator=[1 28.8 400]
  Caracteristique Couple : simulink/Math Operations/Polynomial  coefs="[3.323e-4  -3.102e-2 1.84e-1]"
  Caracteristique Force : simulink/Math Operations/Polynomial  coefs=[2e-5 -1e-3 2e-3]
  Derivative : Derivative
  Gain : Gain  Gain=5000
  Inertie Helice : Gain  Gain=3e-5
  Ki : Gain  Gain=235e-3
  "Nmm -> Nm" : Gain  Gain=1/1000
  RPM vers Rad.s-1 : Gain  Gain=2*pi/60
  "RPM vers Rad.s-1   " : Gain  Gain=2*pi/60
  RPM vers Rad.s-1   1 : Gain  Gain=2*pi/60
  Scope : Scope
      settings: YMin=4990  YMax=5130  SaveName=ScopeData6
  Sum : Sum  Inputs=|++
  T Variateur : TransportDelay  DelayTime=20e-3
  Terminator : Terminator
  Force de poussée : Outport
  Couple : Outport  Port=2
  I consommée : Outport  Port=3
  Omega hélice : Outport  Port=4
  wires:
  Vent relatif/1 -> Terminator/1
  Consigne poussée/1 -> Gain/1
  Caracteristique Force/1 -> Force de poussée/1
  T Variateur/1 -> Asservissement moteur/1
  Asservissement moteur/1 -> Omega hélice/1, RPM vers Rad.s-1   1/1, "RPM vers Rad.s-1   "/1, RPM vers Rad.s-1/1, Scope/1
  Derivative/1 -> Inertie Helice/1
  Caracteristique Couple/1 -> "Nmm -> Nm"/1
  Sum/1 -> Ki/1, Couple/1
  Inertie Helice/1 -> Sum/2
  Ki/1 -> I consommée/1
  Gain/1 -> T Variateur/1
  RPM vers Rad.s-1/1 -> Caracteristique Force/1
  "RPM vers Rad.s-1   "/1 -> Caracteristique Couple/1
  "Nmm -> Nm"/1 -> Sum/1
  RPM vers Rad.s-1   1/1 -> Derivative/1

== system Simulation/Drone/Bras2/ Couple orientation ==
  Omega bras : Inport  Port=1  LatchInput=off
  Derivative1 : Derivative
  Gain : Gain
  Couple orientation : Outport
  wires:
  Omega bras/1 -> Derivative1/1
  Derivative1/1 -> Gain/1
  Gain/1 -> Couple orientation/1

== system Simulation/Drone/Bras2/Couple gyroscopique ==
  Omega helice : Inport  Port=1  LatchInput=off
  Omega bras : Inport  Port=2  LatchInput=off
  Gain : Gain  Gain=[0 27e-6 0]
  Product : Product  RndMeth=Zero
  Couple gyroscopique : Outport
  wires:
  Omega helice/1 -> Product/1
  Omega bras/1 -> Product/2
  Product/1 -> Gain/1
  Gain/1 -> Couple gyroscopique/1

== system Simulation/Drone/Bras2/Matrice rotation couple ==
  Couple entrée : Inport  Port=1  LatchInput=off
  Angle orientation : Inport  Port=2  LatchInput=off
  Constant : Constant  Value=0
  Cos : Trigonometry  Operator=cos
  Gain : Gain  Gain=[ 1 1 -1 ]
  Mux : Mux  Inputs=3
  Product : Product  RndMeth=Zero
  Reshape : simulink/Math Operations/Reshape  OutputDimensionality=1-D array  OutputDimensions=[1,1]
  Sin : Trigonometry
  Couple : Outport
  wires:
  Angle orientation/1 -> Cos/1, Sin/1
  Constant/1 -> Mux/1
  Cos/1 -> Mux/3
  Sin/1 -> Mux/2
  Mux/1 -> Reshape/1
  Gain/1 -> Product/1
  Couple entrée/1 -> Product/2
  Product/1 -> Couple/1
  Reshape/1 -> Gain/1

== system Simulation/Drone/Bras2/Matrice rotation force ==
  Force poussée : Inport  Port=1  LatchInput=off
  Angle orientation : Inport  Port=2  LatchInput=off
  Constant : Constant  Value=0
  Cos : Trigonometry  Operator=cos
  Gain : Gain  Gain=[ 1 1 -1 ]
  Mux : Mux  Inputs=3
  Product : Product  RndMeth=Zero
  Reshape : simulink/Math Operations/Reshape  OutputDimensionality=1-D array  OutputDimensions=[1,1]
  Sin : Trigonometry
  Force : Outport
  wires:
  Angle orientation/1 -> Cos/1, Sin/1
  Constant/1 -> Mux/1
  Cos/1 -> Mux/3
  Sin/1 -> Mux/2
  Mux/1 -> Reshape/1
  Gain/1 -> Product/1
  Force poussée/1 -> Product/2
  Product/1 -> Force/1
  Reshape/1 -> Gain/1

== system Simulation/Drone/Bras2/Servo ==
  Consigne orientation : Inport  Port=1  LatchInput=off
  Temps de réponse orientation1 : TransferFcn  Denominator=[ 0.002 0.05 1]
  Angle orientation : Outport
  wires:
  Consigne orientation/1 -> Temps de réponse orientation1/1
  Temps de réponse orientation1/1 -> Angle orientation/1

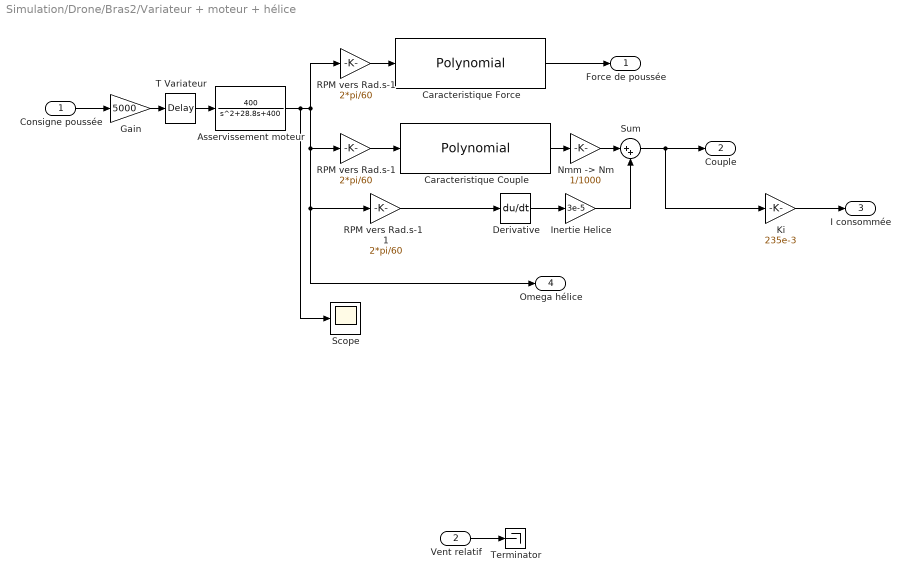
== system Simulation/Drone/Bras2/Variateur + moteur + hélice ==
  Consigne poussée : Inport  Port=1  LatchInput=off
  Vent relatif : Inport  Port=2  LatchInput=off
  Asservissement moteur : TransferFcn  Numerator=[400]  Denominator=[1 28.8 400]
  Caracteristique Couple : simulink/Math Operations/Polynomial  coefs="[3.323e-4  -3.102e-2 1.84e-1]"
  Caracteristique Force : simulink/Math Operations/Polynomial  coefs=[2e-5 -1e-3 2e-3]
  Derivative : Derivative
  Gain : Gain  Gain=5000
  Inertie Helice : Gain  Gain=3e-5
  Ki : Gain  Gain=235e-3
  "Nmm -> Nm" : Gain  Gain=1/1000
  RPM vers Rad.s-1 : Gain  Gain=2*pi/60
  "RPM vers Rad.s-1   " : Gain  Gain=2*pi/60
  RPM vers Rad.s-1   1 : Gain  Gain=2*pi/60
  Scope : Scope
      settings: YMin=4990  YMax=5130  SaveName=ScopeData6
  Sum : Sum  Inputs=|++
  T Variateur : TransportDelay  DelayTime=20e-3
  Terminator : Terminator
  Force de poussée : Outport
  Couple : Outport  Port=2
  I consommée : Outport  Port=3
  Omega hélice : Outport  Port=4
  wires:
  Vent relatif/1 -> Terminator/1
  Consigne poussée/1 -> Gain/1
  Caracteristique Force/1 -> Force de poussée/1
  T Variateur/1 -> Asservissement moteur/1
  Asservissement moteur/1 -> Omega hélice/1, RPM vers Rad.s-1   1/1, "RPM vers Rad.s-1   "/1, RPM vers Rad.s-1/1, Scope/1
  Derivative/1 -> Inertie Helice/1
  Caracteristique Couple/1 -> "Nmm -> Nm"/1
  Sum/1 -> Ki/1, Couple/1
  Inertie Helice/1 -> Sum/2
  Ki/1 -> I consommée/1
  Gain/1 -> T Variateur/1
  RPM vers Rad.s-1/1 -> Caracteristique Force/1
  "RPM vers Rad.s-1   "/1 -> Caracteristique Couple/1
  "Nmm -> Nm"/1 -> Sum/1
  RPM vers Rad.s-1   1/1 -> Derivative/1

== system Simulation/Drone/Bras3/ Couple orientation ==
  Omega bras : Inport  Port=1  LatchInput=off
  Derivative1 : Derivative
  Gain : Gain
  Couple orientation : Outport
  wires:
  Omega bras/1 -> Derivative1/1
  Derivative1/1 -> Gain/1
  Gain/1 -> Couple orientation/1

== system Simulation/Drone/Bras3/Couple gyroscopique ==
  Omega helice : Inport  Port=1  LatchInput=off
  Omega bras : Inport  Port=2  LatchInput=off
  Gain : Gain  Gain=[0 27e-6 0]
  Product : Product  RndMeth=Zero
  Couple gyroscopique : Outport
  wires:
  Omega helice/1 -> Product/1
  Omega bras/1 -> Product/2
  Product/1 -> Gain/1
  Gain/1 -> Couple gyroscopique/1

== system Simulation/Drone/Bras3/Matrice rotation couple ==
  Couple entrée : Inport  Port=1  LatchInput=off
  Angle orientation : Inport  Port=2  LatchInput=off
  Constant : Constant  Value=0
  Cos : Trigonometry  Operator=cos
  Gain : Gain  Gain=[ 1 1 -1 ]
  Mux : Mux  Inputs=3
  Product : Product  RndMeth=Zero
  Reshape : simulink/Math Operations/Reshape  OutputDimensionality=1-D array  OutputDimensions=[1,1]
  Sin : Trigonometry
  Couple : Outport
  wires:
  Angle orientation/1 -> Cos/1, Sin/1
  Constant/1 -> Mux/1
  Cos/1 -> Mux/3
  Sin/1 -> Mux/2
  Mux/1 -> Reshape/1
  Gain/1 -> Product/1
  Couple entrée/1 -> Product/2
  Product/1 -> Couple/1
  Reshape/1 -> Gain/1

== system Simulation/Drone/Bras3/Matrice rotation force ==
  Force poussée : Inport  Port=1  LatchInput=off
  Angle orientation : Inport  Port=2  LatchInput=off
  Constant : Constant  Value=0
  Cos : Trigonometry  Operator=cos
  Gain : Gain  Gain=[ 1 1 -1 ]
  Mux : Mux  Inputs=3
  Product : Product  RndMeth=Zero
  Reshape : simulink/Math Operations/Reshape  OutputDimensionality=1-D array  OutputDimensions=[1,1]
  Sin : Trigonometry
  Force : Outport
  wires:
  Angle orientation/1 -> Cos/1, Sin/1
  Constant/1 -> Mux/1
  Cos/1 -> Mux/3
  Sin/1 -> Mux/2
  Mux/1 -> Reshape/1
  Gain/1 -> Product/1
  Force poussée/1 -> Product/2
  Product/1 -> Force/1
  Reshape/1 -> Gain/1

== system Simulation/Drone/Bras3/Servo ==
  Consigne orientation : Inport  Port=1  LatchInput=off
  Temps de réponse orientation1 : TransferFcn  Denominator=[ 0.002 0.05 1]
  Angle orientation : Outport
  wires:
  Consigne orientation/1 -> Temps de réponse orientation1/1
  Temps de réponse orientation1/1 -> Angle orientation/1

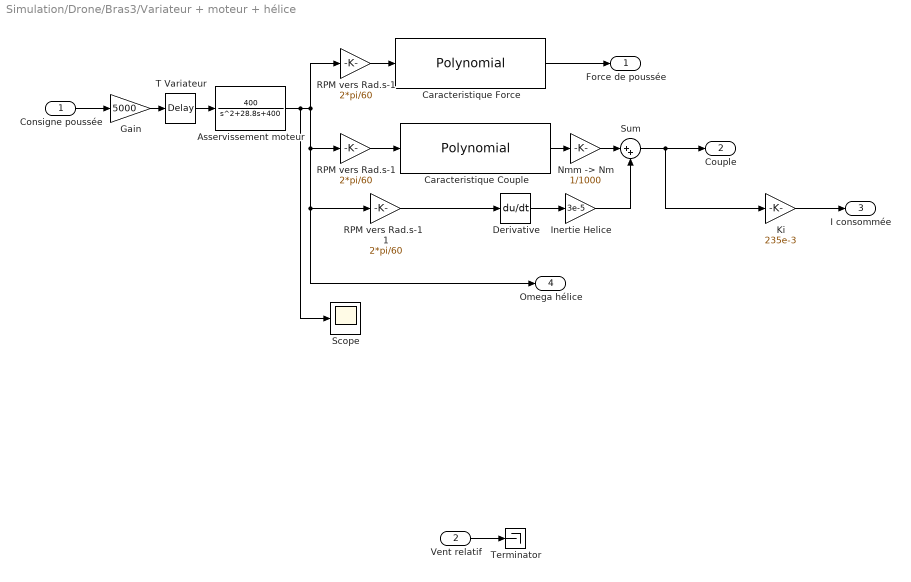
== system Simulation/Drone/Bras3/Variateur + moteur + hélice ==
  Consigne poussée : Inport  Port=1  LatchInput=off
  Vent relatif : Inport  Port=2  LatchInput=off
  Asservissement moteur : TransferFcn  Numerator=[400]  Denominator=[1 28.8 400]
  Caracteristique Couple : simulink/Math Operations/Polynomial  coefs="[3.323e-4  -3.102e-2 1.84e-1]"
  Caracteristique Force : simulink/Math Operations/Polynomial  coefs=[2e-5 -1e-3 2e-3]
  Derivative : Derivative
  Gain : Gain  Gain=5000
  Inertie Helice : Gain  Gain=3e-5
  Ki : Gain  Gain=235e-3
  "Nmm -> Nm" : Gain  Gain=1/1000
  RPM vers Rad.s-1 : Gain  Gain=2*pi/60
  "RPM vers Rad.s-1   " : Gain  Gain=2*pi/60
  RPM vers Rad.s-1   1 : Gain  Gain=2*pi/60
  Scope : Scope
      settings: YMin=4990  YMax=5130  SaveName=ScopeData6
  Sum : Sum  Inputs=|++
  T Variateur : TransportDelay  DelayTime=20e-3
  Terminator : Terminator
  Force de poussée : Outport
  Couple : Outport  Port=2
  I consommée : Outport  Port=3
  Omega hélice : Outport  Port=4
  wires:
  Vent relatif/1 -> Terminator/1
  Consigne poussée/1 -> Gain/1
  Caracteristique Force/1 -> Force de poussée/1
  T Variateur/1 -> Asservissement moteur/1
  Asservissement moteur/1 -> Omega hélice/1, RPM vers Rad.s-1   1/1, "RPM vers Rad.s-1   "/1, RPM vers Rad.s-1/1, Scope/1
  Derivative/1 -> Inertie Helice/1
  Caracteristique Couple/1 -> "Nmm -> Nm"/1
  Sum/1 -> Ki/1, Couple/1
  Inertie Helice/1 -> Sum/2
  Ki/1 -> I consommée/1
  Gain/1 -> T Variateur/1
  RPM vers Rad.s-1/1 -> Caracteristique Force/1
  "RPM vers Rad.s-1   "/1 -> Caracteristique Couple/1
  "Nmm -> Nm"/1 -> Sum/1
  RPM vers Rad.s-1   1/1 -> Derivative/1

== system Simulation/Drone1/Bras1/ Couple orientation ==
  Omega bras : Inport  Port=1  LatchInput=off
  Derivative1 : Derivative
  Gain : Gain
  Couple orientation : Outport
  wires:
  Omega bras/1 -> Derivative1/1
  Derivative1/1 -> Gain/1
  Gain/1 -> Couple orientation/1

== system Simulation/Drone1/Bras1/Couple gyroscopique ==
  Omega helice : Inport  Port=1  LatchInput=off
  Omega bras : Inport  Port=2  LatchInput=off
  Gain : Gain  Gain=[0 27e-6 0]
  Product : Product  RndMeth=Zero
  Couple gyroscopique : Outport
  wires:
  Omega helice/1 -> Product/1
  Omega bras/1 -> Product/2
  Product/1 -> Gain/1
  Gain/1 -> Couple gyroscopique/1

== system Simulation/Drone1/Bras1/Matrice rotation couple ==
  Couple entrée : Inport  Port=1  LatchInput=off
  Angle orientation : Inport  Port=2  LatchInput=off
  Constant : Constant  Value=0
  Cos : Trigonometry  Operator=cos
  Gain : Gain  Gain=[ 1 1 -1 ]
  Mux : Mux  Inputs=3
  Product : Product  RndMeth=Zero
  Reshape : simulink/Math Operations/Reshape  OutputDimensionality=1-D array  OutputDimensions=[1,1]
  Sin : Trigonometry
  Couple : Outport
  wires:
  Angle orientation/1 -> Cos/1, Sin/1
  Constant/1 -> Mux/1
  Cos/1 -> Mux/3
  Sin/1 -> Mux/2
  Mux/1 -> Reshape/1
  Gain/1 -> Product/1
  Couple entrée/1 -> Product/2
  Product/1 -> Couple/1
  Reshape/1 -> Gain/1

== system Simulation/Drone1/Bras1/Matrice rotation force ==
  Force poussée : Inport  Port=1  LatchInput=off
  Angle orientation : Inport  Port=2  LatchInput=off
  Constant : Constant  Value=0
  Cos : Trigonometry  Operator=cos
  Gain : Gain  Gain=[ 1 1 -1 ]
  Mux : Mux  Inputs=3
  Product : Product  RndMeth=Zero
  Reshape : simulink/Math Operations/Reshape  OutputDimensionality=1-D array  OutputDimensions=[1,1]
  Sin : Trigonometry
  Force : Outport
  wires:
  Angle orientation/1 -> Cos/1, Sin/1
  Constant/1 -> Mux/1
  Cos/1 -> Mux/3
  Sin/1 -> Mux/2
  Mux/1 -> Reshape/1
  Gain/1 -> Product/1
  Force poussée/1 -> Product/2
  Product/1 -> Force/1
  Reshape/1 -> Gain/1

== system Simulation/Drone1/Bras1/Servo ==
  Consigne orientation : Inport  Port=1  LatchInput=off
  Temps de réponse orientation1 : TransferFcn  Denominator=[ 0.002 0.05 1]
  Angle orientation : Outport
  wires:
  Consigne orientation/1 -> Temps de réponse orientation1/1
  Temps de réponse orientation1/1 -> Angle orientation/1

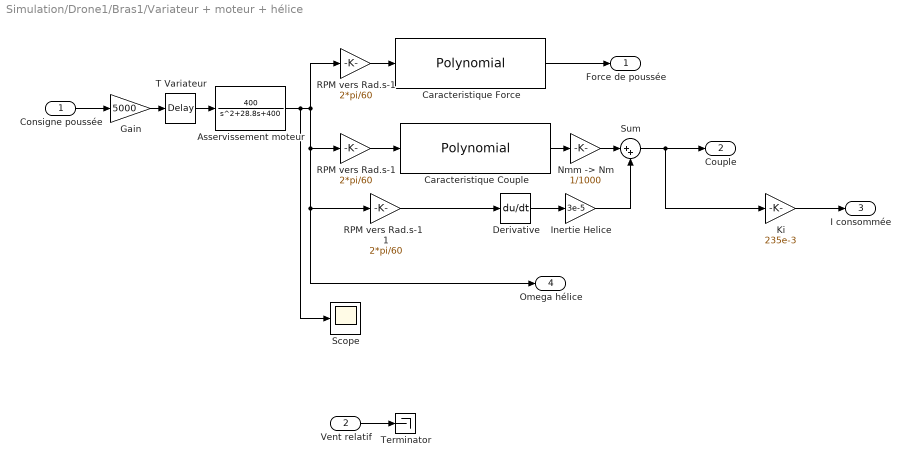
== system Simulation/Drone1/Bras1/Variateur + moteur + hélice ==
  Consigne poussée : Inport  Port=1  LatchInput=off
  Vent relatif : Inport  Port=2  LatchInput=off
  Asservissement moteur : TransferFcn  Numerator=[400]  Denominator=[1 28.8 400]
  Caracteristique Couple : simulink/Math Operations/Polynomial  coefs="[3.323e-4  -3.102e-2 1.84e-1]"
  Caracteristique Force : simulink/Math Operations/Polynomial  coefs=[2e-5 -1e-3 2e-3]
  Derivative : Derivative
  Gain : Gain  Gain=5000
  Inertie Helice : Gain  Gain=3e-5
  Ki : Gain  Gain=235e-3
  "Nmm -> Nm" : Gain  Gain=1/1000
  RPM vers Rad.s-1 : Gain  Gain=2*pi/60
  "RPM vers Rad.s-1   " : Gain  Gain=2*pi/60
  RPM vers Rad.s-1   1 : Gain  Gain=2*pi/60
  Scope : Scope
      settings: YMin=4990  YMax=5130  SaveName=ScopeData6
  Sum : Sum  Inputs=|++
  T Variateur : TransportDelay  DelayTime=20e-3
  Terminator : Terminator
  Force de poussée : Outport
  Couple : Outport  Port=2
  I consommée : Outport  Port=3
  Omega hélice : Outport  Port=4
  wires:
  Vent relatif/1 -> Terminator/1
  Consigne poussée/1 -> Gain/1
  Caracteristique Force/1 -> Force de poussée/1
  T Variateur/1 -> Asservissement moteur/1
  Asservissement moteur/1 -> Omega hélice/1, RPM vers Rad.s-1   1/1, "RPM vers Rad.s-1   "/1, RPM vers Rad.s-1/1, Scope/1
  Derivative/1 -> Inertie Helice/1
  Caracteristique Couple/1 -> "Nmm -> Nm"/1
  Sum/1 -> Ki/1, Couple/1
  Inertie Helice/1 -> Sum/2
  Ki/1 -> I consommée/1
  Gain/1 -> T Variateur/1
  RPM vers Rad.s-1/1 -> Caracteristique Force/1
  "RPM vers Rad.s-1   "/1 -> Caracteristique Couple/1
  "Nmm -> Nm"/1 -> Sum/1
  RPM vers Rad.s-1   1/1 -> Derivative/1

== system Simulation/Subsystem/Controle Bras 1/Adaptation Consigne1 ==
  Force : Inport  Port=1  LatchInput=off
  Constant : Constant  Value=2*a
  Constant1 : Constant  Value=-b
  Constant2 : Constant  Value=c
  Divide : Product  Inputs=*/  OutScaling=2^-10
  Math Function : Math  Operator=sqrt  SaturateOnIntegerOverflow=on
  Polynomial : simulink/Math Operations/Polynomial  coefs=[-4*a b*b]
  Scope : Scope
      settings: YMin=0  YMax=1000  SaveName=ScopeData7
  Subtract : Sum  OutScaling=2^-10
  Subtract1 : Sum  Inputs=-+  OutScaling=2^-10
  Consigne Omega : Outport
  wires:
  Constant/1 -> Divide/2
  Constant1/1 -> Subtract/2
  Subtract/1 -> Divide/1
  Divide/1 -> Consigne Omega/1
  Math Function/1 -> Subtract/1
  Polynomial/1 -> Math Function/1
  Force/1 -> Scope/1, Subtract1/1
  Subtract1/1 -> Polynomial/1
  Constant2/1 -> Subtract1/2

== system Simulation/Subsystem/Controle Bras 1/Controle Bras1 ==
  Fyc : Inport  Port=1  LatchInput=off
  Fzc : Inport  Port=2  LatchInput=off
  Complex to Magnitude-Angle : ComplexToMagnitudeAngle
  Real-Imag to Complex : RealImagToComplex
  Unary Minus : simulink/Math Operations/Unary Minus  DoSatur=off
  Force Propulsion : Outport
  Angle Orientation : Outport  Port=2
  wires:
  Real-Imag to Complex/1 -> Complex to Magnitude-Angle/1
  Complex to Magnitude-Angle/2 -> Angle Orientation/1
  Complex to Magnitude-Angle/1 -> Force Propulsion/1
  Fyc/1 -> Real-Imag to Complex/2
  Fzc/1 -> Unary Minus/1
  Unary Minus/1 -> Real-Imag to Complex/1
